simulink model "paceMakerModel_group10_3"  (R2020a)
settings: Solver=FixedStepAuto  StartTime=0.0  StopTime=10.0  FixedStep=1e-3  RelTol=1e-3  EnableMultiTasking=on
undefined symbols (not defined in the file): A0, A1, D0, D1, D10, D11, D12, D13, D2, D3, D4, D5, D6, D7, D8, D9, PTA0, PTA1, PTA2, PTB2, PTB23, PTB3, PTB9, PTC16, PTC17, PTC2, PTC3, PTC4, PTD0, PTD1, PTD2, PTD3
libraries: frdmk64flib x20, etargetslib x2
settings Model: ExtModeTrigDuration=5  Creator=wxavi  LastModifiedBy=Will
settings OptimizationCC: EnhancedBackFolding=on  PassReuseOutputArgsAs=Individual arguments  ZeroExternalMemoryAtStartup=off  ZeroInternalMemoryAtStartup=off  MaxStackSize=64  OptimizeBlockOrder=speed  DifferentSizesBufferReuse=on  OptimizationCustomize=off  EfficientTunableParamExpr=on
settings DebuggingCC: ParameterTunabilityLossMsg=error
settings HardwareCC: ProdBitPerPointer=32  ProdBitPerSizeT=32  ProdBitPerPtrDiffT=32  ProdLargestAtomicInteger=Long  ProdLargestAtomicFloat=Double  ProdWordSize=32  ProdHWDeviceType=ARM Compatible->ARM Cortex
settings SFSimCC: MATLABDynamicMemAlloc=off
settings RTWCC: SystemTargetFile=ert.tlc  HardwareBoard=NXP FRDM-K64F  TemplateMakefile=ert_default_tmf  Toolchain=GNU Tools for ARM Embedded Processors
settings CodeAppCC: ForceParamTrailComments=on  IgnoreCustomStorageClasses=off  OperatorAnnotations=on  SimulinkDataObjDesc=on  SFDataObjDesc=on  InsertBlockDesc=on

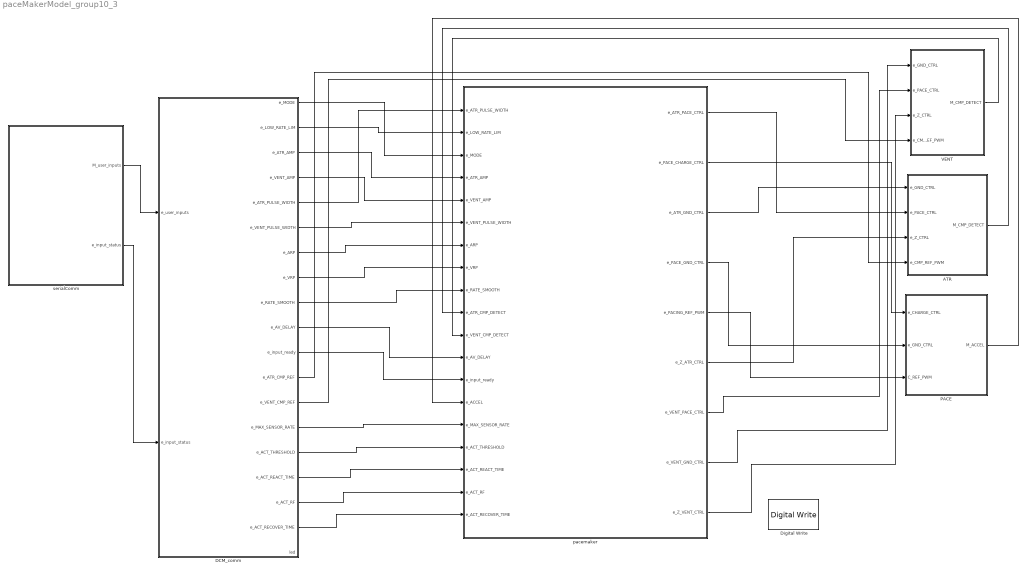
== system paceMakerModel_group10_3 ==
  ATR : Subsystem
  DCM_comm : Stateflow chart  TreatAsAtomicUnit=on
  Digital Write : frdmk64flib/Digital Write  Whichpin=RED_LED
  PACE : Subsystem
  VENT : Subsystem
  pacemaker : Stateflow chart  TreatAsAtomicUnit=on
  serialComm : Subsystem
  wires:
  ATR/1(M_CMP_DETECT) -> pacemaker/10(e_ATR_CMP_DETECT)
  VENT/1(M_CMP_DETECT) -> pacemaker/11(e_VENT_CMP_DETECT)
  pacemaker/1(e_ATR_PACE_CTRL) -> ATR/2(e_PACE_CTRL)
  pacemaker/2(e_PACE_CHARGE_CTRL) -> PACE/1(e_CHARGE_CTRL)
  pacemaker/3(e_ATR_GND_CTRL) -> ATR/1(e_GND_CTRL)
  pacemaker/4(e_PACE_GND_CTRL) -> PACE/2(e_GND_CTRL)
  pacemaker/5(e_PACING_REF_PWM) -> PACE/3(C_REF_PWM)
  pacemaker/6(e_Z_ATR_CTRL) -> ATR/3(e_Z_CTRL)
  pacemaker/7(e_VENT_PACE_CTRL) -> VENT/2(e_PACE_CTRL)
  pacemaker/8(e_VENT_GND_CTRL) -> VENT/1(e_GND_CTRL)
  pacemaker/9(e_Z_VENT_CTRL) -> VENT/3(e_Z_CTRL)
  serialComm/1(M_user_inputs) -> DCM_comm/1(e_user_inputs)
  serialComm/2(e_input_status) -> DCM_comm/2(e_input_status)
  DCM_comm/11(e_input_ready) -> pacemaker/13(e_input_ready)
  DCM_comm/1(e_MODE) -> pacemaker/3(e_MODE)
  DCM_comm/2(e_LOW_RATE_LIM) -> pacemaker/2(e_LOW_RATE_LIM)
  DCM_comm/3(e_ATR_AMP) -> pacemaker/4(e_ATR_AMP)
  DCM_comm/4(e_VENT_AMP) -> pacemaker/5(e_VENT_AMP)
  DCM_comm/5(e_ATR_PULSE_WIDTH) -> pacemaker/1(e_ATR_PULSE_WIDTH)
  DCM_comm/6(e_VENT_PULSE_WIDTH) -> pacemaker/6(e_VENT_PULSE_WIDTH)
  DCM_comm/7(e_ARP) -> pacemaker/7(e_ARP)
  DCM_comm/8(e_VRP) -> pacemaker/8(e_VRP)
  DCM_comm/9(e_RATE_SMOOTH) -> pacemaker/9(e_RATE_SMOOTH)
  DCM_comm/10(e_AV_DELAY) -> pacemaker/12(e_AV_DELAY)
  DCM_comm/12(e_ATR_CMP_REF) -> ATR/4(e_CMP_REF_PWM)
  DCM_comm/13(e_VENT_CMP_REF) -> VENT/4(e_CMP_REF_PWM)
  PACE/1(M_ACCEL) -> pacemaker/14(e_ACCEL)
  DCM_comm/14(e_MAX_SENSOR_RATE) -> pacemaker/15(e_MAX_SENSOR_RATE)
  DCM_comm/18(e_ACT_RECOVER_TIME) -> pacemaker/19(e_ACT_RECOVER_TIME)
  DCM_comm/17(e_ACT_RF) -> pacemaker/18(e_ACT_RF)
  DCM_comm/16(e_ACT_REACT_TIME) -> pacemaker/17(e_ACT_REACT_TIME)
  DCM_comm/15(e_ACT_THRESHOLD) -> pacemaker/16(e_ACT_THRESHOLD)
  ? -> Digital Write/1

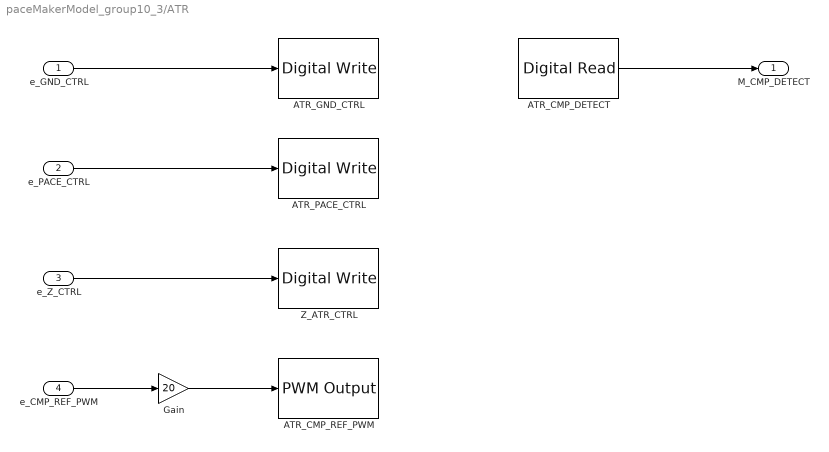
== system paceMakerModel_group10_3/ATR ==
  e_GND_CTRL : Inport
  e_PACE_CTRL : Inport  Port=2
  e_Z_CTRL : Inport  Port=3
  e_CMP_REF_PWM : Inport  Port=4
  ATR_CMP_DETECT : frdmk64flib/Digital Read  Whichpin=PTC16 (D0)  SampleTime=-1
  ATR_CMP_REF_PWM : frdmk64flib/PWM Output  Whichpin=PTC2 (D6)  InitialFrequency=2000  InitialDutyCycle=0
  ATR_GND_CTRL : frdmk64flib/Digital Write  Whichpin=PTD2 (D11)
  ATR_PACE_CTRL : frdmk64flib/Digital Write  Whichpin=PTA0 (D8)
  Gain : Gain  Gain=20
  Z_ATR_CTRL : frdmk64flib/Digital Write  Whichpin=PTB23 (D4)
  M_CMP_DETECT : Outport
  wires:
  e_Z_CTRL/1 -> Z_ATR_CTRL/1
  e_GND_CTRL/1 -> ATR_GND_CTRL/1
  e_PACE_CTRL/1 -> ATR_PACE_CTRL/1
  e_CMP_REF_PWM/1 -> Gain/1
  ATR_CMP_DETECT/1 -> M_CMP_DETECT/1
  Gain/1 -> ATR_CMP_REF_PWM/1

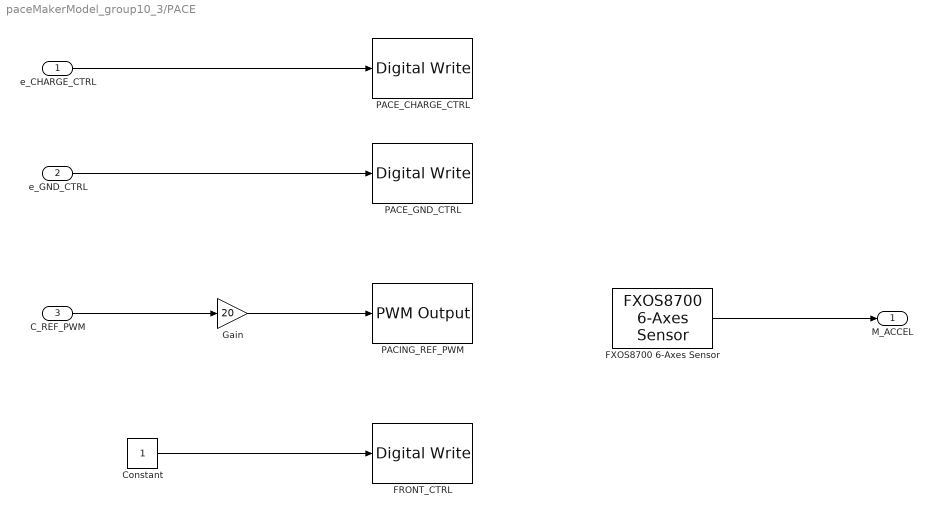
== system paceMakerModel_group10_3/PACE ==
  e_CHARGE_CTRL : Inport
  e_GND_CTRL : Inport  Port=2
  C_REF_PWM : Inport  Port=3
  Constant : Constant
  FRONT_CTRL : frdmk64flib/Digital Write  Whichpin=PTD1 (D13)
  FXOS8700 6-Axes Sensor : frdmk64flib/FXOS8700 6-Axes Sensor  Activesensor=Accelerometer only  ODR=100Hz  HybridODR=100Hz  Accelfullrange=-4g to +4g  SampleTime=-1
  Gain : Gain  Gain=20
  PACE_CHARGE_CTRL : frdmk64flib/Digital Write  Whichpin=PTB9 (D2)
  PACE_GND_CTRL : frdmk64flib/Digital Write  Whichpin=PTD0 (D10)
  PACING_REF_PWM : frdmk64flib/PWM Output  Whichpin=PTA2 (D5)  InitialFrequency=2000  InitialDutyCycle=0
  M_ACCEL : Outport
  wires:
  Gain/1 -> PACING_REF_PWM/1
  C_REF_PWM/1 -> Gain/1
  e_GND_CTRL/1 -> PACE_GND_CTRL/1
  e_CHARGE_CTRL/1 -> PACE_CHARGE_CTRL/1
  Constant/1 -> FRONT_CTRL/1
  FXOS8700 6-Axes Sensor/1 -> M_ACCEL/1

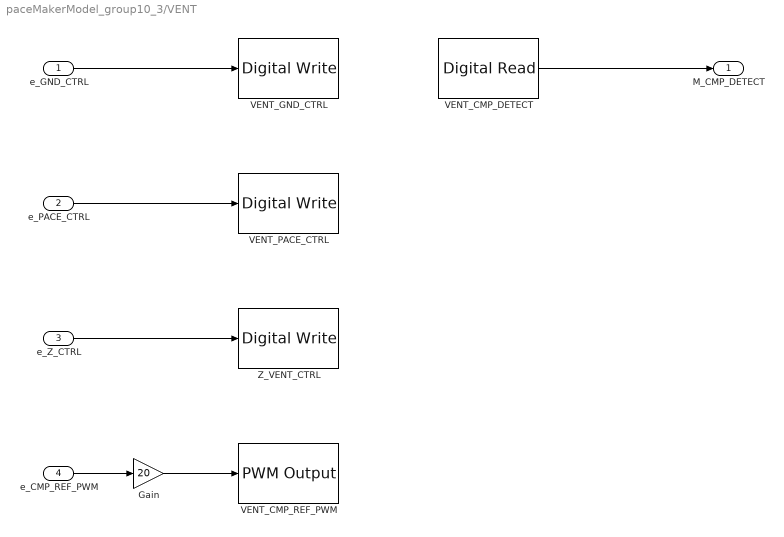
== system paceMakerModel_group10_3/VENT ==
  e_GND_CTRL : Inport
  e_PACE_CTRL : Inport  Port=2
  e_Z_CTRL : Inport  Port=3
  e_CMP_REF_PWM : Inport  Port=4
  Gain : Gain  Gain=20
  VENT_CMP_DETECT : frdmk64flib/Digital Read  Whichpin=PTC17 (D1)  SampleTime=-1
  VENT_CMP_REF_PWM : frdmk64flib/PWM Output  Whichpin=PTA1 (D3)  InitialFrequency=2000  InitialDutyCycle=0
  VENT_GND_CTRL : frdmk64flib/Digital Write  Whichpin=PTD3 (D12)
  VENT_PACE_CTRL : frdmk64flib/Digital Write  Whichpin=PTC4 (D9)
  Z_VENT_CTRL : frdmk64flib/Digital Write  Whichpin=PTC3 (D7)
  M_CMP_DETECT : Outport
  wires:
  e_GND_CTRL/1 -> VENT_GND_CTRL/1
  e_PACE_CTRL/1 -> VENT_PACE_CTRL/1
  e_Z_CTRL/1 -> Z_VENT_CTRL/1
  e_CMP_REF_PWM/1 -> Gain/1
  VENT_CMP_DETECT/1 -> M_CMP_DETECT/1
  Gain/1 -> VENT_CMP_REF_PWM/1

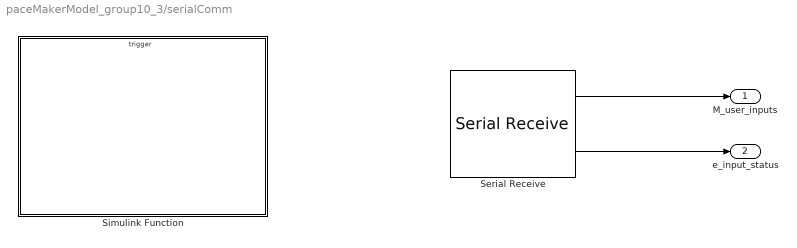
== system paceMakerModel_group10_3/serialComm ==
  Serial Receive : frdmk64flib/Serial Receive  SCIModule=0  Baudrate=uint32(9600)  Parity=None  StopBits=1  HardwareFlowControl=None  ByteOrder=LittleEndian  DataType=uint8  DataLength=54  BlockingMode=off  OutputStatus=on  SampleTime=-1
  Simulink Function : Subsystem  TreatAsAtomicUnit=on
  M_user_inputs : Outport
  e_input_status : Outport  Port=2
  wires:
  Serial Receive/2 -> e_input_status/1
  Serial Receive/1 -> M_user_inputs/1

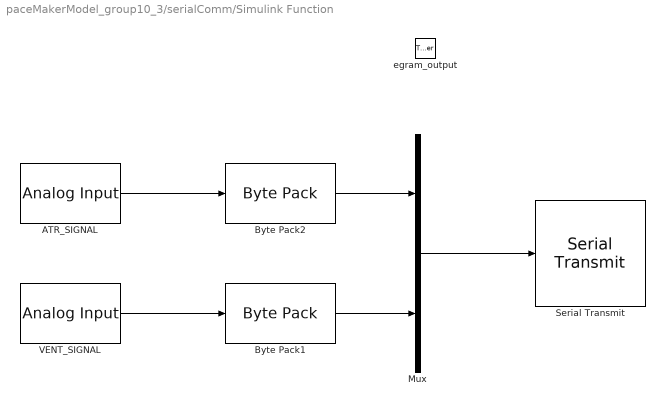
== system paceMakerModel_group10_3/serialComm/Simulink Function ==
  egram_output : TriggerPort  TriggerType=function-call  IsSimulinkFunction=on  FunctionName=egram_output  VariantControl=(inherit)
  ATR_SIGNAL : frdmk64flib/Analog Input  Whichpin=PTB2 (A0)  SampleTime=-1
  Byte Pack1 : etargetslib/Byte Pack  datatypes={'double'}  byteAlign=1
  Byte Pack2 : etargetslib/Byte Pack  datatypes={'double'}  byteAlign=1
  Mux : Mux  Inputs=2
  Serial Transmit : frdmk64flib/Serial Transmit  SCIModule=0  Baudrate=uint32(9600)  Parity=None  StopBits=1  HardwareFlowControl=None  ByteOrder=LittleEndian  BlockingMode=on  OutputStatus=off
  VENT_SIGNAL : frdmk64flib/Analog Input  Whichpin=PTB3 (A1)  SampleTime=-1
  wires:
  Byte Pack1/1 -> Mux/2
  Mux/1 -> Serial Transmit/1
  Byte Pack2/1 -> Mux/1
  VENT_SIGNAL/1 -> Byte Pack1/1
  ATR_SIGNAL/1 -> Byte Pack2/1

== stateflow chart paceMakerModel_group10_3/DCM_comm ==
  state send_egram
    entry:
    e_send_req = e_user_inputs(1);
    e_MODE = e_user_inputs(2);
    e_LOW_RATE_LIM = typecast(e_user_inputs(3:4),'int16');
    e_ATR_AMP = typecast(e_user_inputs(5:8),'single');
    e_VENT_AMP = typecast(e_user_inputs(9:12),'single');
    e_ATR_PULSE_WIDTH = typecast(e_user_inputs(13:20),'double');
    e_VENT_PULSE_WIDTH = typecast(e_user_inputs(21:28),'double');
    e_ARP = typecast(e_user_inputs(29:30),'int16');
    e_VRP = typecast(e_user_inputs(31:32),'int16');
    e_RATE_SMOOTH = typecast(e_user_inputs(33:40),'double');
    e_AV_DELAY = typecast(e_user_inputs(41:42),'int16');
    e_ATR_CMP_REF = e_user_inputs(43);
    e_VENT_CMP_REF = e_user_inputs(44);
    e_MAX_SENSOR_RATE = typecast(e_user_inputs(45:46),'int16');;
    e_ACT_THRESHOLD = typecast(e_user_inputs(47:48),'int16');;
    e_ACT_REACT_TIME = typecast(e_user_inputs(49:50),'int16');;
    e_ACT_RF = typecast(e_user_inputs(51:52),'int16');;
    e_ACT_RECOVER_TIME = typecast(e_user_inputs(53:54),'int16');
    if (e_send_req) egram_output();
    else e_input_ready = 1; end
  state comm_init
    entry:
    led = 0;
  state status_check
    entry:
    e_input_ready = 0;
  (default) -> comm_init
  status_check -> send_egram : [~e_input_status]
  comm_init -> status_check
  send_egram -> status_check
  data: e_user_inputs input uint8; e_input_status input uint8; e_MODE output uint8; e_LOW_RATE_LIM output int16; e_ATR_AMP output single; e_VENT_AMP output single; e_ATR_PULSE_WIDTH output double; e_VENT_PULSE_WIDTH output double; e_ARP output int16; e_VRP output int16; e_RATE_SMOOTH output double; e_AV_DELAY output int16; e_input_ready output uint8; e_ATR_CMP_REF output uint8; e_VENT_CMP_REF output uint8; e_MAX_SENSOR_RATE output int16; e_ACT_THRESHOLD output int16; e_ACT_REACT_TIME output int16; e_ACT_RF output int16; e_ACT_RECOVER_TIME output int16; led output int8; e_send_req local uint8

== stateflow chart paceMakerModel_group10_3/pacemaker ==
  settings: executeAtInitialization=1
  state RATE_MODULATION
    entry:
    switch e_accel_rec_count
    case 1
    e_accel_rec_1 = abs(e_ACCEL(1)) + abs(e_ACCEL(2));
    case 2
    e_accel_rec_2 =  abs(e_ACCEL(1)) + abs(e_ACCEL(2));
    case 3
    e_accel_rec_3 = abs(e_ACCEL(1)) + abs(e_ACCEL(2));
    case 4
    e_accel_rec_4 = abs(e_ACCEL(1)) + abs(e_ACCEL(2)) ;
    end
    if (e_accel_rec_count >= 4)
    e_accel_rec_count = 1;
    else
    e_accel_rec_count = e_accel_rec_count + 1;
    end
    e_act_level = 20*((e_accel_rec_1 + e_accel_rec_2 + e_accel_rec_3 + e_accel_rec_4)/4 - 0.1);
    if (e_act_level >e_ACT_THRESHOLD)
    e_rm_rate = int16(double(e_LOW_RATE_LIM) + double(((e_act_level - e_ACT_THRESHOLD)*(e_MAX_SENSOR_RATE - e_LOW_RATE_LIM)/(40-2*e_ACT_RF))));
    e_rm_duration =int16(double(e_ACT_REACT_TIME)*(e_rm_rate - double(e_LOW_RATE_LIM))/double(e_MAX_SENSOR_RATE - e_LOW_RATE_LIM));
    e_PULSE_INT = 60000/((int16(e_rm_rate - double(e_LOW_RATE_LIM))*e_PULSE_INT/(1000*e_rm_duration)) + 60000/e_PULSE_INT);
    if (60000/e_PULSE_INT > e_MAX_SENSOR_RATE)
    e_PULSE_INT = 60000/e_MAX_SENSOR_RATE;
    end
    else
    if (60000/e_PULSE_INT > e_LOW_RATE_LIM)
    e_PULSE_INT = int16(double(60000/((60000/double(e_PULSE_INT))-(double(e_MAX_SENSOR_RATE - e_LOW_RATE_LIM)*double(e_PULSE_INT)/double(e_ACT_RECOVER_TIME*1000)))));
    end
    end
  state MODE_CHECK
    entry:
    e_PULSE_INT = 60/e_LOW_RATE_LIM*1000;
    if (e_MODE == 0 || e_MODE == 2 || e_MODE == 10 || e_MODE == 12)
    e_PULSE_WIDTH = e_ATR_PULSE_WIDTH;
    e_PULSE_AMP = e_ATR_AMP;
    else
    e_PULSE_WIDTH = e_VENT_PULSE_WIDTH;
    e_PULSE_AMP = e_VENT_AMP;
    end
    e_PACING_REF_PWM = e_PULSE_AMP;
    if (e_MODE == 2 || e_MODE == 3 || e_MODE == 12 || e_MODE == 13)
    e_PULSE_INT = e_PULSE_INT * e_RATE_SMOOTH;
    end
    e_accel_rec_count = 1;
    e_accel_rec_1 = 0;
    e_accel_rec_2 = 0;
    e_accel_rec_3 = 0;
    e_accel_rec_4 = 0;
    e_rm_rate = e_LOW_RATE_LIM;
  state A_Charge
    entry:
    e_PACE_CHARGE_CTRL = 1;
    e_ATR_GND_CTRL = 1;
    e_ATR_PACE_CTRL = 0;
    e_PACE_GND_CTRL = 1;
    e_VENT_PACE_CTRL = 0;
    e_VENT_GND_CTRL = 0;
    e_Z_ATR_CTRL = 0;
    e_Z_VENT_CTRL = 0;
  state V_Charge
    entry:
    e_PACE_CHARGE_CTRL = 1;
    e_VENT_GND_CTRL = 1;
    e_VENT_PACE_CTRL = 0;
    e_PACE_GND_CTRL = 1;
    e_ATR_PACE_CTRL = 0;
    e_ATR_GND_CTRL = 0;
    e_Z_ATR_CTRL = 0;
    e_Z_VENT_CTRL = 0;
  state V_SENSE
  state A_SENSE
  state V_Pace
    entry:
    e_PACE_CHARGE_CTRL = 0;
    e_VENT_GND_CTRL = 0;
    e_VENT_PACE_CTRL = 1;
  state A_Pace
    entry:
    e_PACE_CHARGE_CTRL = 0;
    e_ATR_GND_CTRL = 0;
    e_ATR_PACE_CTRL = 1;
  RATE_MODULATION -> A_Charge [order 1] : [e_MODE == 10 || e_MODE == 12 || e_MODE == 14]
  RATE_MODULATION -> V_Charge [order 2] : [e_MODE == 11 || e_MODE == 13]
  V_Pace -> RATE_MODULATION [order 4] : [ (e_MODE == 11 || e_MODE == 13 || e_MODE == 14) && after(e_PULSE_WIDTH,msec)]
  A_Pace -> RATE_MODULATION [order 4] : [(e_MODE == 10 || e_MODE == 12) && after(e_PULSE_WIDTH,msec)]
  (default) -> MODE_CHECK
  MODE_CHECK -> A_Charge [order 1] : [e_MODE == 0 || e_MODE == 2 || e_MODE == 4 || e_MODE == 10 || e_MODE == 12 || e_MODE == 14]
  MODE_CHECK -> V_Charge [order 2] : [e_MODE == 1 || e_MODE == 3 || e_MODE == 11 || e_MODE == 13]
  A_Charge -> MODE_CHECK [order 4] : [e_input_ready]
  V_Charge -> MODE_CHECK [order 4] : [e_input_ready]
  A_SENSE -> A_Charge [order 2] : [e_ATR_CMP_DETECT]
  V_SENSE -> V_Charge [order 1] : [e_VENT_CMP_DETECT]
  A_SENSE -> MODE_CHECK [order 3] : [e_input_ready]
  A_Charge -> A_SENSE [order 1] : [after(e_ARP,msec) && (e_MODE == 2 || e_MODE == 12)]
  V_Charge -> V_SENSE [order 1] : [after(e_VRP,msec)&& (e_MODE == 3 || e_MODE == 13)]
  V_SENSE -> MODE_CHECK [order 3] : [e_input_ready]
  V_Pace -> A_Charge [order 2] : [(e_MODE == 4) && after(e_VENT_PULSE_WIDTH,msec)]
  A_Pace -> V_Charge [order 2] : [(e_MODE ==4|| e_MODE == 14) && after(e_ATR_PULSE_WIDTH,msec)]
  V_Charge -> V_Pace [order 2] : [(e_MODE == 1 || e_MODE == 11) && after(e_PULSE_INT - e_PULSE_WIDTH,msec)]
  V_Pace -> V_Charge [order 1] : [(e_MODE == 1 || e_MODE == 3) && after(e_PULSE_WIDTH,msec)]
  V_Charge -> V_Pace [order 3] : [(e_MODE ==4 || e_MODE == 14) && after(e_AV_DELAY,msec)]
  V_Pace -> MODE_CHECK [order 3] : [e_input_ready]
  A_Pace -> MODE_CHECK [order 3] : [e_input_ready]
  A_Charge -> A_Pace [order 3] : [(e_MODE == 4 || e_MODE == 14) && after(e_PULSE_INT - e_ATR_PULSE_WIDTH-e_VENT_PULSE_WIDTH -e_AV_DELAY,msec)]
  A_Charge -> A_Pace [order 2] : [(e_MODE == 0 || e_MODE == 10) &&after(e_PULSE_INT - e_PULSE_WIDTH,msec) ]
  A_Pace -> A_Charge [order 1] : [(e_MODE == 0 || e_MODE == 2) && after(e_PULSE_WIDTH,msec)]
  V_SENSE -> V_Pace [order 2] : [after(e_PULSE_INT - e_PULSE_WIDTH-e_VRP,msec) && ~e_VENT_CMP_DETECT]
  A_SENSE -> A_Pace [order 1] : [after(e_PULSE_INT-e_PULSE_WIDTH-e_ARP,msec) && ~e_ATR_CMP_DETECT]
  data: e_ATR_PULSE_WIDTH input double; e_ATR_PACE_CTRL output int16; e_PACE_CHARGE_CTRL output int16; e_ATR_GND_CTRL output int16; e_LOW_RATE_LIM input int16; e_MODE input uint8; e_ATR_AMP input single; e_VENT_AMP input single; e_VENT_PULSE_WIDTH input double; e_PACE_GND_CTRL output int16; e_PACING_REF_PWM output single; e_Z_ATR_CTRL output int16; e_VENT_PACE_CTRL output int16; e_VENT_GND_CTRL output int16; e_Z_VENT_CTRL output int16; e_ARP input int16; e_VRP input int16; e_RATE_SMOOTH input double; e_ATR_CMP_DETECT input boolean; e_VENT_CMP_DETECT input boolean; e_PULSE_WIDTH local double; e_PULSE_INT local int16; e_PULSE_AMP local single; e_AV_DELAY input int16; e_input_ready input uint8; e_ACCEL input double; e_MAX_SENSOR_RATE input int16; e_ACT_THRESHOLD input int16; e_ACT_REACT_TIME input int16; e_ACT_RF input int16; e_ACT_RECOVER_TIME input int16; e_act_level local double; e_rm_rate local int16; e_rm_duration local int16; e_accel_rec_count local int8; e_accel_rec_1 local double; e_accel_rec_2 local double; e_accel_rec_3 local double; e_accel_rec_4 local double
